simulink model "HarmonicDecay_TestModel"  (R2014a)
settings: Solver=ode8  StartTime=0.0  StopTime=10.0  FixedStep=0.01  RelTol=1e-3
libraries: rocket_angular_flight_library x1
settings Model: Creator=scorpii  LastModifiedBy=scorpii

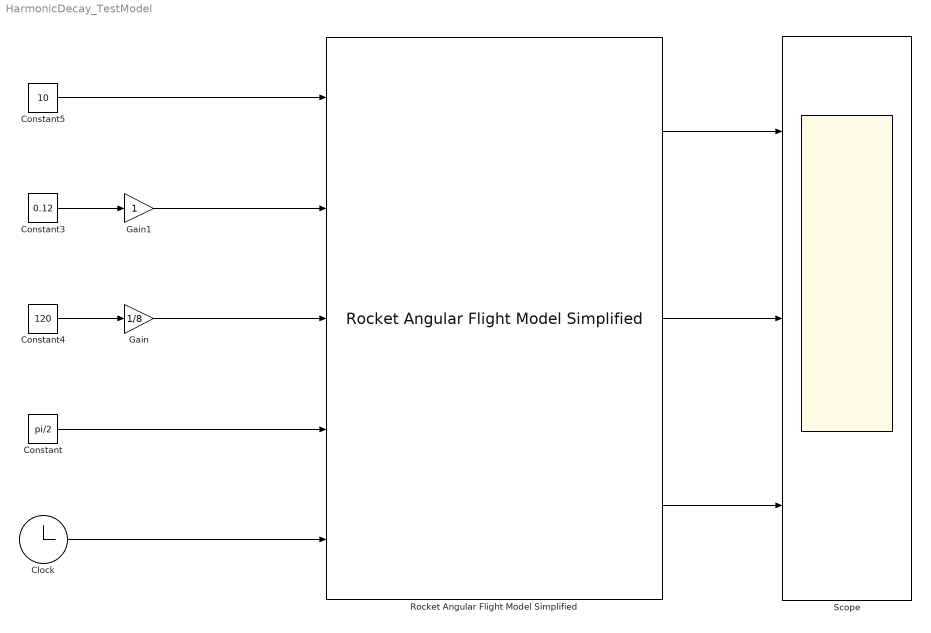
== system HarmonicDecay_TestModel ==
  Clock : Clock
  Constant : Constant  Value=pi/2
  Constant3 : Constant  Value=0.12
  Constant4 : Constant  Value=120
  Constant5 : Constant  Value=10
  Gain : Gain  Gain=1/8
  Gain1 : Gain
  Rocket Angular Flight Model Simplified : rocket_angular_flight_library/Rocket Angular Flight Model Simplified  SystemSampleTime=-1
  Scope : Scope  NumInputPorts=3
      settings: YMin=-5~-5~-5  YMax=5~5~5
  wires:
  Clock/1 -> Rocket Angular Flight Model Simplified/5
  Rocket Angular Flight Model Simplified/1 -> Scope/1
  Constant4/1 -> Gain/1
  Rocket Angular Flight Model Simplified/2 -> Scope/2
  Rocket Angular Flight Model Simplified/3 -> Scope/3
  Constant3/1 -> Gain1/1
  Constant5/1 -> Rocket Angular Flight Model Simplified/1
  Constant/1 -> Rocket Angular Flight Model Simplified/4
  Gain1/1 -> Rocket Angular Flight Model Simplified/2
  Gain/1 -> Rocket Angular Flight Model Simplified/3
